simulink model "rmspec"  (Simulink 7.0)
settings: Solver=ode45  StartTime=0.0  StopTime=200  RelTol=1e-3
undefined symbols (not defined in the file): pfb_coeff_gen_calc
libraries: xbsIndex_r4 x3092, casper_library x230, xps_library x24
(part 32 of 33)

== system rmspec/pfb/fft_wideband_real1/fft_biplex_real_4x0/biplex_core/fft_stage_9/butterfly_direct/twiddle/coeff_gen ==
  rst : Inport
  Counter : xbsIndex_r4/Counter  cnt_type=Free Running  cnt_to=Inf  operation=Up  start_count=0  cnt_by_val=1  arith_type=Unsigned  n_bits=8  bin_pt=0  load_pin=off  rst=on  en=off  explicit_period=on  period=1  dbl_ovrd=off  use_behavioral_HDL=off  use_rpm=off  implementation=Fabric  block_type=counter
  ROM : xbsIndex_r4/ROM  depth=256  initVector=[1 0 0.707107543945313 -0.707107543945313 0.923881530761719 -0.382682800292969 0.382682800292969 -0.923881530761719 0.980781555175781 -0.195091247558594 0.555572509765625 -0.831466674804688 0.831466674804688 -0.555572509765625 0.195091247558594 -0.980781555175781 0.995185852050781 -0.0980148315429688 0.634391784667969 -0.77301025390625 0.881919860839844 -0.471397399902344 0.290283203125 -0.956939697265625 0.956939697265625 -0.290283203125 0.471397399902344 -0.881919860839844 0.77301025390625 -0.634391784667969 0.0980148315429688 -0.995185852050781 0.998794555664063 -0.0490646362304688 0.671562194824219 -0.740951538085938 0.90399169921875 -0.427558898925781 0.336891174316406 -0.941543579101563 0.97003173828125 -0.24298095703125 0.51409912109375 -0.85772705078125 0.803207397460938 -0.595695495605469 0.146728515625 -0.989173889160156 0.989173889160156 -0.146728515625 0.595695495605469 -0.803207397460938 0.85772705078125 -0.51409912109375 0.24298095703125 -0.97003173828125 0.941543579101563 -0.336891174316406 0.427558898925781 -0.90399169921875 0.740951538085938 -0.671562194824219 0.0490646362304688 -0.998794555664063 0.999702453613281 -0.0245437622070313 0.689537048339844 -0.724250793457031 0.914207458496094 -0.405242919921875 0.359893798828125 -0.932991027832031 0.975700378417969 -0.219100952148438 0.534996032714844 -0.844856262207031 0.817581176757813 -0.5758056640625 0.17095947265625 -0.985275268554688 0.992477416992188 -0.122413635253906 0.615234375 -0.788345336914063 0.870086669921875 -0.492897033691406 0.266716003417969 -0.963775634765625 0.949531555175781 -0.313682556152344 0.449607849121094 -0.893226623535156 0.757209777832031 -0.653175354003906 0.0735626220703125 -0.997291564941406 0.997291564941406 -0.0735626220703125 0.653175354003906 -0.757209777832031 0.893226623535156 -0.449607849121094 0.313682556152344 -0.949531555175781 0.963775634765625 -0.266716003417969 0.492897033691406 -0.870086669921875 0.788345336914063 -0.615234375 0.122413635253906 -0.992477416992188 0.985275268554688 -0.17095947265625 0.5758056640625 -0.817581176757813 0.844856262207031 -0.534996032714844 0.219100952148438 -0.975700378417969 0.932991027832031 -0.359893798828125 0.405242919921875 -0.914207458496094 0.724250793457031 -0.689537048339844 0.0245437622070313 -0.999702453613281 0.999923706054688 -0.01226806640625 0.698379516601563 -0.715728759765625 0.919113159179688 -0.393989562988281 0.371315002441406 -0.928504943847656 0.978317260742188 -0.207115173339844 0.545326232910156 -0.838226318359375 0.824592590332031 -0.56573486328125 0.183036804199219 -0.983108520507813 0.993904113769531 -0.110221862792969 0.624862670898438 -0.780738830566406 0.876068115234375 -0.482185363769531 0.278518676757813 -0.960433959960938 0.95330810546875 -0.302009582519531 0.460540771484375 -0.887641906738281 0.765167236328125 -0.643829345703125 0.0858001708984375 -0.996315002441406 0.998115539550781 -0.0613174438476563 0.66241455078125 -0.749137878417969 0.898674011230469 -0.438613891601563 0.325309753417969 -0.945610046386719 0.96697998046875 -0.254867553710938 0.5035400390625 -0.863975524902344 0.79583740234375 -0.605514526367188 0.13458251953125 -0.99090576171875 0.9873046875 -0.158859252929688 0.585800170898438 -0.810455322265625 0.851356506347656 -0.524589538574219 0.231056213378906 -0.972938537597656 0.937339782714844 -0.348419189453125 0.416427612304688 -0.909164428710938 0.732650756835938 -0.68060302734375 0.03680419921875 -0.999320983886719 0.999320983886719 -0.03680419921875 0.68060302734375 -0.732650756835938 0.909164428710938 -0.416427612304688 0.348419189453125 -0.937339782714844 0.972938537597656 -0.231056213378906 0.524589538574219 -0.851356506347656 0.810455322265625 -0.585800170898438 0.158859252929688 -0.9873046875 0.99090576171875 -0.13458251953125 0.605514526367188 -0.79583740234375 0.863975524902344 -0.5035400390625 0.254867553710938 -0.96697998046875 0.945610046386719 -0.325309753417969 0.438613891601563 -0.898674011230469 0.749137878417969 ...(+646 chars)]  distributed_mem=Block RAM  rst=off  init_reg=0  en=off  latency=2  arith_type="Signed  (2's comp)"  n_bits=18  bin_pt=17  dbl_ovrd=off  optimize=Area  use_rpm=on  block_type=sprom
      settings: block_version=10.1.3
  ROM1 : xbsIndex_r4/ROM  depth=256  initVector=[0 -1 -0.707107543945313 -0.707107543945313 -0.382682800292969 -0.923881530761719 -0.923881530761719 -0.382682800292969 -0.195091247558594 -0.980781555175781 -0.831466674804688 -0.555572509765625 -0.555572509765625 -0.831466674804688 -0.980781555175781 -0.195091247558594 -0.0980148315429688 -0.995185852050781 -0.77301025390625 -0.634391784667969 -0.471397399902344 -0.881919860839844 -0.956939697265625 -0.290283203125 -0.290283203125 -0.956939697265625 -0.881919860839844 -0.471397399902344 -0.634391784667969 -0.77301025390625 -0.995185852050781 -0.0980148315429688 -0.0490646362304688 -0.998794555664063 -0.740951538085938 -0.671562194824219 -0.427558898925781 -0.90399169921875 -0.941543579101563 -0.336891174316406 -0.24298095703125 -0.97003173828125 -0.85772705078125 -0.51409912109375 -0.595695495605469 -0.803207397460938 -0.989173889160156 -0.146728515625 -0.146728515625 -0.989173889160156 -0.803207397460938 -0.595695495605469 -0.51409912109375 -0.85772705078125 -0.97003173828125 -0.24298095703125 -0.336891174316406 -0.941543579101563 -0.90399169921875 -0.427558898925781 -0.671562194824219 -0.740951538085938 -0.998794555664063 -0.0490646362304688 -0.0245437622070313 -0.999702453613281 -0.724250793457031 -0.689537048339844 -0.405242919921875 -0.914207458496094 -0.932991027832031 -0.359893798828125 -0.219100952148438 -0.975700378417969 -0.844856262207031 -0.534996032714844 -0.5758056640625 -0.817581176757813 -0.985275268554688 -0.17095947265625 -0.122413635253906 -0.992477416992188 -0.788345336914063 -0.615234375 -0.492897033691406 -0.870086669921875 -0.963775634765625 -0.266716003417969 -0.313682556152344 -0.949531555175781 -0.893226623535156 -0.449607849121094 -0.653175354003906 -0.757209777832031 -0.997291564941406 -0.0735626220703125 -0.0735626220703125 -0.997291564941406 -0.757209777832031 -0.653175354003906 -0.449607849121094 -0.893226623535156 -0.949531555175781 -0.313682556152344 -0.266716003417969 -0.963775634765625 -0.870086669921875 -0.492897033691406 -0.615234375 -0.788345336914063 -0.992477416992188 -0.122413635253906 -0.17095947265625 -0.985275268554688 -0.817581176757813 -0.5758056640625 -0.534996032714844 -0.844856262207031 -0.975700378417969 -0.219100952148438 -0.359893798828125 -0.932991027832031 -0.914207458496094 -0.405242919921875 -0.689537048339844 -0.724250793457031 -0.999702453613281 -0.0245437622070313 -0.01226806640625 -0.999923706054688 -0.715728759765625 -0.698379516601563 -0.393989562988281 -0.919113159179688 -0.928504943847656 -0.371315002441406 -0.207115173339844 -0.978317260742188 -0.838226318359375 -0.545326232910156 -0.56573486328125 -0.824592590332031 -0.983108520507813 -0.183036804199219 -0.110221862792969 -0.993904113769531 -0.780738830566406 -0.624862670898438 -0.482185363769531 -0.876068115234375 -0.960433959960938 -0.278518676757813 -0.302009582519531 -0.95330810546875 -0.887641906738281 -0.460540771484375 -0.643829345703125 -0.765167236328125 -0.996315002441406 -0.0858001708984375 -0.0613174438476563 -0.998115539550781 -0.749137878417969 -0.66241455078125 -0.438613891601563 -0.898674011230469 -0.945610046386719 -0.325309753417969 -0.254867553710938 -0.96697998046875 -0.863975524902344 -0.5035400390625 -0.605514526367188 -0.79583740234375 -0.99090576171875 -0.13458251953125 -0.158859252929688 -0.9873046875 -0.810455322265625 -0.585800170898438 -0.524589538574219 -0.851356506347656 -0.972938537597656 -0.231056213378906 -0.348419189453125 -0.937339782714844 -0.909164428710938 -0.416427612304688 -0.68060302734375 -0.732650756835938 -0.999320983886719 -0.03680419921875 -0.03680419921875 -0.999320983886719 -0.732650756835938 -0.68060302734375 -0.416427612304688 -0.909164428710938 -0.937339782714844 -0.348419189453125 -0.231056213378906 -0.972938537597656 -0.851356506347656 -0.524589538574219 -0.585800170898438 -0.810455322265625 -0.9873046875 -0.158859252929688 -0.13458251953125 -0.99090576171875 -0.79583740234375 -0.605514526367188 -0.5035400390625 -0.863975524902344 -0.96697998046875 ...(+777 chars)]  distributed_mem=Block RAM  rst=off  init_reg=0  en=off  latency=2  arith_type="Signed  (2's comp)"  n_bits=18  bin_pt=17  dbl_ovrd=off  optimize=Area  use_rpm=on  block_type=sprom
      settings: block_version=10.1.3
  Slice : xbsIndex_r4/Slice  nbits=8  boolean_output=off  mode=Upper Bit Location + Width  bit1=0  base1=MSB of Input  bit0=0  base0=LSB of Input  dbl_ovrd=off  block_type=slice
      settings: infoedit="Extracts a given range of bits from each input sample and presents it at the output.  The output type is ordinarily unsigned with binary point at zero, but can be Boolean when the slice is one bit wide.<P><P>Hardware notes: In hardware this block costs nothing."  block_version=10.1.3
  ri_to_c : casper_library/Misc/ri_to_c  SystemSampleTime=-1
  w : Outport
  wires:
  ri_to_c/1 -> w/1
  rst/1 -> Counter/1
  Counter/1 -> Slice/1
  Slice/1 -> ROM/1, ROM1/1
  ROM/1 -> ri_to_c/1
  ROM1/1 -> ri_to_c/2

== system rmspec/pfb/fft_wideband_real1/fft_biplex_real_4x0/biplex_core/fft_stage_9/butterfly_direct/twiddle/convert_of ==
  din : Inport  OutDataType=sfix(16)  OutScaling=2^0
  convert : xbsIndex_r4/Convert  arith_type="Signed  (2's comp)"  n_bits=bit_width_o  bin_pt=binary_point_o  quantization=Truncate  overflow=Wrap  latency=latency  dbl_ovrd=off  pipeline=on  block_type=convert
      settings: block_version=10.1.1
  never : xbsIndex_r4/Constant  arith_type=Boolean  const=0  n_bits=16  bin_pt=14  explicit_period=on  period=1  equ=P=C  opselect=C  inp2=PCIN>>17  opr=+  inp1=P  carry=CIN  dbl_ovrd=off  block_type=constant
  dout : Outport
  of : Outport  Port=2
  wires:
  din/1 -> convert/1
  convert/1 -> dout/1
  never/1 -> of/1

== system rmspec/pfb/fft_wideband_real1/fft_biplex_real_4x0/biplex_core/fft_stage_9/butterfly_direct/twiddle/convert_of1 ==
  din : Inport  OutDataType=sfix(16)  OutScaling=2^0
  convert : xbsIndex_r4/Convert  arith_type="Signed  (2's comp)"  n_bits=bit_width_o  bin_pt=binary_point_o  quantization=Truncate  overflow=Wrap  latency=latency  dbl_ovrd=off  pipeline=on  block_type=convert
      settings: block_version=10.1.1
  never : xbsIndex_r4/Constant  arith_type=Boolean  const=0  n_bits=16  bin_pt=14  explicit_period=on  period=1  equ=P=C  opselect=C  inp2=PCIN>>17  opr=+  inp1=P  carry=CIN  dbl_ovrd=off  block_type=constant
  dout : Outport
  of : Outport  Port=2
  wires:
  din/1 -> convert/1
  convert/1 -> dout/1
  never/1 -> of/1

== system rmspec/w_fft/fft/fft_biplex0/biplex_core/fft_stage_10/butterfly_direct/twiddle/coeff_gen ==
  rst : Inport
  Counter : xbsIndex_r4/Counter  cnt_type=Free Running  cnt_to=Inf  operation=Up  start_count=0  cnt_by_val=1  arith_type=Unsigned  n_bits=9  bin_pt=0  load_pin=off  rst=on  en=off  explicit_period=on  period=1  dbl_ovrd=off  use_behavioral_HDL=off  use_rpm=off  implementation=Fabric  block_type=counter
  ROM : xbsIndex_r4/ROM  depth=512  initVector=[1 0 0.707107543945313 -0.707107543945313 0.923881530761719 -0.382682800292969 0.382682800292969 -0.923881530761719 0.980781555175781 -0.195091247558594 0.555572509765625 -0.831466674804688 0.831466674804688 -0.555572509765625 0.195091247558594 -0.980781555175781 0.995185852050781 -0.0980148315429688 0.634391784667969 -0.77301025390625 0.881919860839844 -0.471397399902344 0.290283203125 -0.956939697265625 0.956939697265625 -0.290283203125 0.471397399902344 -0.881919860839844 0.77301025390625 -0.634391784667969 0.0980148315429688 -0.995185852050781 0.998794555664063 -0.0490646362304688 0.671562194824219 -0.740951538085938 0.90399169921875 -0.427558898925781 0.336891174316406 -0.941543579101563 0.97003173828125 -0.24298095703125 0.51409912109375 -0.85772705078125 0.803207397460938 -0.595695495605469 0.146728515625 -0.989173889160156 0.989173889160156 -0.146728515625 0.595695495605469 -0.803207397460938 0.85772705078125 -0.51409912109375 0.24298095703125 -0.97003173828125 0.941543579101563 -0.336891174316406 0.427558898925781 -0.90399169921875 0.740951538085938 -0.671562194824219 0.0490646362304688 -0.998794555664063 0.999702453613281 -0.0245437622070313 0.689537048339844 -0.724250793457031 0.914207458496094 -0.405242919921875 0.359893798828125 -0.932991027832031 0.975700378417969 -0.219100952148438 0.534996032714844 -0.844856262207031 0.817581176757813 -0.5758056640625 0.17095947265625 -0.985275268554688 0.992477416992188 -0.122413635253906 0.615234375 -0.788345336914063 0.870086669921875 -0.492897033691406 0.266716003417969 -0.963775634765625 0.949531555175781 -0.313682556152344 0.449607849121094 -0.893226623535156 0.757209777832031 -0.653175354003906 0.0735626220703125 -0.997291564941406 0.997291564941406 -0.0735626220703125 0.653175354003906 -0.757209777832031 0.893226623535156 -0.449607849121094 0.313682556152344 -0.949531555175781 0.963775634765625 -0.266716003417969 0.492897033691406 -0.870086669921875 0.788345336914063 -0.615234375 0.122413635253906 -0.992477416992188 0.985275268554688 -0.17095947265625 0.5758056640625 -0.817581176757813 0.844856262207031 -0.534996032714844 0.219100952148438 -0.975700378417969 0.932991027832031 -0.359893798828125 0.405242919921875 -0.914207458496094 0.724250793457031 -0.689537048339844 0.0245437622070313 -0.999702453613281 0.999923706054688 -0.01226806640625 0.698379516601563 -0.715728759765625 0.919113159179688 -0.393989562988281 0.371315002441406 -0.928504943847656 0.978317260742188 -0.207115173339844 0.545326232910156 -0.838226318359375 0.824592590332031 -0.56573486328125 0.183036804199219 -0.983108520507813 0.993904113769531 -0.110221862792969 0.624862670898438 -0.780738830566406 0.876068115234375 -0.482185363769531 0.278518676757813 -0.960433959960938 0.95330810546875 -0.302009582519531 0.460540771484375 -0.887641906738281 0.765167236328125 -0.643829345703125 0.0858001708984375 -0.996315002441406 0.998115539550781 -0.0613174438476563 0.66241455078125 -0.749137878417969 0.898674011230469 -0.438613891601563 0.325309753417969 -0.945610046386719 0.96697998046875 -0.254867553710938 0.5035400390625 -0.863975524902344 0.79583740234375 -0.605514526367188 0.13458251953125 -0.99090576171875 0.9873046875 -0.158859252929688 0.585800170898438 -0.810455322265625 0.851356506347656 -0.524589538574219 0.231056213378906 -0.972938537597656 0.937339782714844 -0.348419189453125 0.416427612304688 -0.909164428710938 0.732650756835938 -0.68060302734375 0.03680419921875 -0.999320983886719 0.999320983886719 -0.03680419921875 0.68060302734375 -0.732650756835938 0.909164428710938 -0.416427612304688 0.348419189453125 -0.937339782714844 0.972938537597656 -0.231056213378906 0.524589538574219 -0.851356506347656 0.810455322265625 -0.585800170898438 0.158859252929688 -0.9873046875 0.99090576171875 -0.13458251953125 0.605514526367188 -0.79583740234375 0.863975524902344 -0.5035400390625 0.254867553710938 -0.96697998046875 0.945610046386719 -0.325309753417969 0.438613891601563 -0.898674011230469 0.749137878417969 ...(+5316 chars)]  distributed_mem=Block RAM  rst=off  init_reg=0  en=off  latency=2  arith_type="Signed  (2's comp)"  n_bits=18  bin_pt=17  dbl_ovrd=off  optimize=Area  use_rpm=on  block_type=sprom
      settings: block_version=10.1.3
  ROM1 : xbsIndex_r4/ROM  depth=512  initVector=[0 -1 -0.707107543945313 -0.707107543945313 -0.382682800292969 -0.923881530761719 -0.923881530761719 -0.382682800292969 -0.195091247558594 -0.980781555175781 -0.831466674804688 -0.555572509765625 -0.555572509765625 -0.831466674804688 -0.980781555175781 -0.195091247558594 -0.0980148315429688 -0.995185852050781 -0.77301025390625 -0.634391784667969 -0.471397399902344 -0.881919860839844 -0.956939697265625 -0.290283203125 -0.290283203125 -0.956939697265625 -0.881919860839844 -0.471397399902344 -0.634391784667969 -0.77301025390625 -0.995185852050781 -0.0980148315429688 -0.0490646362304688 -0.998794555664063 -0.740951538085938 -0.671562194824219 -0.427558898925781 -0.90399169921875 -0.941543579101563 -0.336891174316406 -0.24298095703125 -0.97003173828125 -0.85772705078125 -0.51409912109375 -0.595695495605469 -0.803207397460938 -0.989173889160156 -0.146728515625 -0.146728515625 -0.989173889160156 -0.803207397460938 -0.595695495605469 -0.51409912109375 -0.85772705078125 -0.97003173828125 -0.24298095703125 -0.336891174316406 -0.941543579101563 -0.90399169921875 -0.427558898925781 -0.671562194824219 -0.740951538085938 -0.998794555664063 -0.0490646362304688 -0.0245437622070313 -0.999702453613281 -0.724250793457031 -0.689537048339844 -0.405242919921875 -0.914207458496094 -0.932991027832031 -0.359893798828125 -0.219100952148438 -0.975700378417969 -0.844856262207031 -0.534996032714844 -0.5758056640625 -0.817581176757813 -0.985275268554688 -0.17095947265625 -0.122413635253906 -0.992477416992188 -0.788345336914063 -0.615234375 -0.492897033691406 -0.870086669921875 -0.963775634765625 -0.266716003417969 -0.313682556152344 -0.949531555175781 -0.893226623535156 -0.449607849121094 -0.653175354003906 -0.757209777832031 -0.997291564941406 -0.0735626220703125 -0.0735626220703125 -0.997291564941406 -0.757209777832031 -0.653175354003906 -0.449607849121094 -0.893226623535156 -0.949531555175781 -0.313682556152344 -0.266716003417969 -0.963775634765625 -0.870086669921875 -0.492897033691406 -0.615234375 -0.788345336914063 -0.992477416992188 -0.122413635253906 -0.17095947265625 -0.985275268554688 -0.817581176757813 -0.5758056640625 -0.534996032714844 -0.844856262207031 -0.975700378417969 -0.219100952148438 -0.359893798828125 -0.932991027832031 -0.914207458496094 -0.405242919921875 -0.689537048339844 -0.724250793457031 -0.999702453613281 -0.0245437622070313 -0.01226806640625 -0.999923706054688 -0.715728759765625 -0.698379516601563 -0.393989562988281 -0.919113159179688 -0.928504943847656 -0.371315002441406 -0.207115173339844 -0.978317260742188 -0.838226318359375 -0.545326232910156 -0.56573486328125 -0.824592590332031 -0.983108520507813 -0.183036804199219 -0.110221862792969 -0.993904113769531 -0.780738830566406 -0.624862670898438 -0.482185363769531 -0.876068115234375 -0.960433959960938 -0.278518676757813 -0.302009582519531 -0.95330810546875 -0.887641906738281 -0.460540771484375 -0.643829345703125 -0.765167236328125 -0.996315002441406 -0.0858001708984375 -0.0613174438476563 -0.998115539550781 -0.749137878417969 -0.66241455078125 -0.438613891601563 -0.898674011230469 -0.945610046386719 -0.325309753417969 -0.254867553710938 -0.96697998046875 -0.863975524902344 -0.5035400390625 -0.605514526367188 -0.79583740234375 -0.99090576171875 -0.13458251953125 -0.158859252929688 -0.9873046875 -0.810455322265625 -0.585800170898438 -0.524589538574219 -0.851356506347656 -0.972938537597656 -0.231056213378906 -0.348419189453125 -0.937339782714844 -0.909164428710938 -0.416427612304688 -0.68060302734375 -0.732650756835938 -0.999320983886719 -0.03680419921875 -0.03680419921875 -0.999320983886719 -0.732650756835938 -0.68060302734375 -0.416427612304688 -0.909164428710938 -0.937339782714844 -0.348419189453125 -0.231056213378906 -0.972938537597656 -0.851356506347656 -0.524589538574219 -0.585800170898438 -0.810455322265625 -0.9873046875 -0.158859252929688 -0.13458251953125 -0.99090576171875 -0.79583740234375 -0.605514526367188 -0.5035400390625 -0.863975524902344 -0.96697998046875 ...(+5575 chars)]  distributed_mem=Block RAM  rst=off  init_reg=0  en=off  latency=2  arith_type="Signed  (2's comp)"  n_bits=18  bin_pt=17  dbl_ovrd=off  optimize=Area  use_rpm=on  block_type=sprom
      settings: block_version=10.1.3
  Slice : xbsIndex_r4/Slice  nbits=9  boolean_output=off  mode=Upper Bit Location + Width  bit1=0  base1=MSB of Input  bit0=0  base0=LSB of Input  dbl_ovrd=off  block_type=slice
      settings: infoedit="Extracts a given range of bits from each input sample and presents it at the output.  The output type is ordinarily unsigned with binary point at zero, but can be Boolean when the slice is one bit wide.<P><P>Hardware notes: In hardware this block costs nothing."  block_version=10.1.3
  ri_to_c : casper_library/Misc/ri_to_c  SystemSampleTime=-1
  w : Outport
  wires:
  ri_to_c/1 -> w/1
  rst/1 -> Counter/1
  Counter/1 -> Slice/1
  Slice/1 -> ROM/1, ROM1/1
  ROM/1 -> ri_to_c/1
  ROM1/1 -> ri_to_c/2

== system rmspec/w_fft/fft/fft_biplex0/biplex_core/fft_stage_10/butterfly_direct/twiddle/convert_of ==
  din : Inport  OutDataType=sfix(16)  OutScaling=2^0
  convert : xbsIndex_r4/Convert  arith_type="Signed  (2's comp)"  n_bits=bit_width_o  bin_pt=binary_point_o  quantization=Truncate  overflow=Wrap  latency=latency  dbl_ovrd=off  pipeline=on  block_type=convert
      settings: block_version=10.1.1
  never : xbsIndex_r4/Constant  arith_type=Boolean  const=0  n_bits=16  bin_pt=14  explicit_period=on  period=1  equ=P=C  opselect=C  inp2=PCIN>>17  opr=+  inp1=P  carry=CIN  dbl_ovrd=off  block_type=constant
  dout : Outport
  of : Outport  Port=2
  wires:
  din/1 -> convert/1
  convert/1 -> dout/1
  never/1 -> of/1

== system rmspec/w_fft/fft/fft_biplex0/biplex_core/fft_stage_10/butterfly_direct/twiddle/convert_of1 ==
  din : Inport  OutDataType=sfix(16)  OutScaling=2^0
  convert : xbsIndex_r4/Convert  arith_type="Signed  (2's comp)"  n_bits=bit_width_o  bin_pt=binary_point_o  quantization=Truncate  overflow=Wrap  latency=latency  dbl_ovrd=off  pipeline=on  block_type=convert
      settings: block_version=10.1.1
  never : xbsIndex_r4/Constant  arith_type=Boolean  const=0  n_bits=16  bin_pt=14  explicit_period=on  period=1  equ=P=C  opselect=C  inp2=PCIN>>17  opr=+  inp1=P  carry=CIN  dbl_ovrd=off  block_type=constant
  dout : Outport
  of : Outport  Port=2
  wires:
  din/1 -> convert/1
  convert/1 -> dout/1
  never/1 -> of/1

== system rmspec/w_fft/fft/fft_biplex0/biplex_core/fft_stage_3/butterfly_direct/twiddle/coeff_gen ==
  rst : Inport
  Counter : xbsIndex_r4/Counter  cnt_type=Free Running  cnt_to=Inf  operation=Up  start_count=0  cnt_by_val=1  arith_type=Unsigned  n_bits=9  bin_pt=0  load_pin=off  rst=on  en=off  explicit_period=on  period=1  dbl_ovrd=off  use_behavioral_HDL=off  use_rpm=off  implementation=Fabric  block_type=counter
  ROM : xbsIndex_r4/ROM  depth=4  initVector=[1 0 0.707107543945313 -0.707107543945313]  distributed_mem=Distributed memory  rst=off  init_reg=0  en=off  latency=2  arith_type="Signed  (2's comp)"  n_bits=18  bin_pt=17  dbl_ovrd=off  optimize=Area  use_rpm=on  block_type=sprom
      settings: block_version=10.1.3
  ROM1 : xbsIndex_r4/ROM  depth=4  initVector=[0 -1 -0.707107543945313 -0.707107543945313]  distributed_mem=Distributed memory  rst=off  init_reg=0  en=off  latency=2  arith_type="Signed  (2's comp)"  n_bits=18  bin_pt=17  dbl_ovrd=off  optimize=Area  use_rpm=on  block_type=sprom
      settings: block_version=10.1.3
  Slice : xbsIndex_r4/Slice  nbits=2  boolean_output=off  mode=Upper Bit Location + Width  bit1=0  base1=MSB of Input  bit0=0  base0=LSB of Input  dbl_ovrd=off  block_type=slice
      settings: infoedit="Extracts a given range of bits from each input sample and presents it at the output.  The output type is ordinarily unsigned with binary point at zero, but can be Boolean when the slice is one bit wide.<P><P>Hardware notes: In hardware this block costs nothing."  block_version=10.1.3
  ri_to_c : casper_library/Misc/ri_to_c  SystemSampleTime=-1
  w : Outport
  wires:
  ri_to_c/1 -> w/1
  rst/1 -> Counter/1
  Counter/1 -> Slice/1
  Slice/1 -> ROM/1, ROM1/1
  ROM/1 -> ri_to_c/1
  ROM1/1 -> ri_to_c/2

== system rmspec/w_fft/fft/fft_biplex0/biplex_core/fft_stage_3/butterfly_direct/twiddle/convert_of ==
  din : Inport  OutDataType=sfix(16)  OutScaling=2^0
  convert : xbsIndex_r4/Convert  arith_type="Signed  (2's comp)"  n_bits=bit_width_o  bin_pt=binary_point_o  quantization=Truncate  overflow=Wrap  latency=latency  dbl_ovrd=off  pipeline=on  block_type=convert
      settings: block_version=10.1.1
  never : xbsIndex_r4/Constant  arith_type=Boolean  const=0  n_bits=16  bin_pt=14  explicit_period=on  period=1  equ=P=C  opselect=C  inp2=PCIN>>17  opr=+  inp1=P  carry=CIN  dbl_ovrd=off  block_type=constant
  dout : Outport
  of : Outport  Port=2
  wires:
  din/1 -> convert/1
  convert/1 -> dout/1
  never/1 -> of/1

== system rmspec/w_fft/fft/fft_biplex0/biplex_core/fft_stage_3/butterfly_direct/twiddle/convert_of1 ==
  din : Inport  OutDataType=sfix(16)  OutScaling=2^0
  convert : xbsIndex_r4/Convert  arith_type="Signed  (2's comp)"  n_bits=bit_width_o  bin_pt=binary_point_o  quantization=Truncate  overflow=Wrap  latency=latency  dbl_ovrd=off  pipeline=on  block_type=convert
      settings: block_version=10.1.1
  never : xbsIndex_r4/Constant  arith_type=Boolean  const=0  n_bits=16  bin_pt=14  explicit_period=on  period=1  equ=P=C  opselect=C  inp2=PCIN>>17  opr=+  inp1=P  carry=CIN  dbl_ovrd=off  block_type=constant
  dout : Outport
  of : Outport  Port=2
  wires:
  din/1 -> convert/1
  convert/1 -> dout/1
  never/1 -> of/1

== system rmspec/w_fft/fft/fft_biplex0/biplex_core/fft_stage_4/butterfly_direct/twiddle/coeff_gen ==
  rst : Inport
  Counter : xbsIndex_r4/Counter  cnt_type=Free Running  cnt_to=Inf  operation=Up  start_count=0  cnt_by_val=1  arith_type=Unsigned  n_bits=9  bin_pt=0  load_pin=off  rst=on  en=off  explicit_period=on  period=1  dbl_ovrd=off  use_behavioral_HDL=off  use_rpm=off  implementation=Fabric  block_type=counter
  ROM : xbsIndex_r4/ROM  depth=8  initVector=[1 0 0.707107543945313 -0.707107543945313 0.923881530761719 -0.382682800292969 0.382682800292969 -0.923881530761719]  distributed_mem=Distributed memory  rst=off  init_reg=0  en=off  latency=2  arith_type="Signed  (2's comp)"  n_bits=18  bin_pt=17  dbl_ovrd=off  optimize=Area  use_rpm=on  block_type=sprom
      settings: block_version=10.1.3
  ROM1 : xbsIndex_r4/ROM  depth=8  initVector=[0 -1 -0.707107543945313 -0.707107543945313 -0.382682800292969 -0.923881530761719 -0.923881530761719 -0.382682800292969]  distributed_mem=Distributed memory  rst=off  init_reg=0  en=off  latency=2  arith_type="Signed  (2's comp)"  n_bits=18  bin_pt=17  dbl_ovrd=off  optimize=Area  use_rpm=on  block_type=sprom
      settings: block_version=10.1.3
  Slice : xbsIndex_r4/Slice  nbits=3  boolean_output=off  mode=Upper Bit Location + Width  bit1=0  base1=MSB of Input  bit0=0  base0=LSB of Input  dbl_ovrd=off  block_type=slice
      settings: infoedit="Extracts a given range of bits from each input sample and presents it at the output.  The output type is ordinarily unsigned with binary point at zero, but can be Boolean when the slice is one bit wide.<P><P>Hardware notes: In hardware this block costs nothing."  block_version=10.1.3
  ri_to_c : casper_library/Misc/ri_to_c  SystemSampleTime=-1
  w : Outport
  wires:
  ri_to_c/1 -> w/1
  rst/1 -> Counter/1
  Counter/1 -> Slice/1
  Slice/1 -> ROM/1, ROM1/1
  ROM/1 -> ri_to_c/1
  ROM1/1 -> ri_to_c/2

== system rmspec/w_fft/fft/fft_biplex0/biplex_core/fft_stage_4/butterfly_direct/twiddle/convert_of ==
  din : Inport  OutDataType=sfix(16)  OutScaling=2^0
  convert : xbsIndex_r4/Convert  arith_type="Signed  (2's comp)"  n_bits=bit_width_o  bin_pt=binary_point_o  quantization=Truncate  overflow=Wrap  latency=latency  dbl_ovrd=off  pipeline=on  block_type=convert
      settings: block_version=10.1.1
  never : xbsIndex_r4/Constant  arith_type=Boolean  const=0  n_bits=16  bin_pt=14  explicit_period=on  period=1  equ=P=C  opselect=C  inp2=PCIN>>17  opr=+  inp1=P  carry=CIN  dbl_ovrd=off  block_type=constant
  dout : Outport
  of : Outport  Port=2
  wires:
  din/1 -> convert/1
  convert/1 -> dout/1
  never/1 -> of/1

== system rmspec/w_fft/fft/fft_biplex0/biplex_core/fft_stage_4/butterfly_direct/twiddle/convert_of1 ==
  din : Inport  OutDataType=sfix(16)  OutScaling=2^0
  convert : xbsIndex_r4/Convert  arith_type="Signed  (2's comp)"  n_bits=bit_width_o  bin_pt=binary_point_o  quantization=Truncate  overflow=Wrap  latency=latency  dbl_ovrd=off  pipeline=on  block_type=convert
      settings: block_version=10.1.1
  never : xbsIndex_r4/Constant  arith_type=Boolean  const=0  n_bits=16  bin_pt=14  explicit_period=on  period=1  equ=P=C  opselect=C  inp2=PCIN>>17  opr=+  inp1=P  carry=CIN  dbl_ovrd=off  block_type=constant
  dout : Outport
  of : Outport  Port=2
  wires:
  din/1 -> convert/1
  convert/1 -> dout/1
  never/1 -> of/1

== system rmspec/w_fft/fft/fft_biplex0/biplex_core/fft_stage_5/butterfly_direct/twiddle/coeff_gen ==
  rst : Inport
  Counter : xbsIndex_r4/Counter  cnt_type=Free Running  cnt_to=Inf  operation=Up  start_count=0  cnt_by_val=1  arith_type=Unsigned  n_bits=9  bin_pt=0  load_pin=off  rst=on  en=off  explicit_period=on  period=1  dbl_ovrd=off  use_behavioral_HDL=off  use_rpm=off  implementation=Fabric  block_type=counter
  ROM : xbsIndex_r4/ROM  depth=16  initVector=[1 0 0.707107543945313 -0.707107543945313 0.923881530761719 -0.382682800292969 0.382682800292969 -0.923881530761719 0.980781555175781 -0.195091247558594 0.555572509765625 -0.831466674804688 0.831466674804688 -0.555572509765625 0.195091247558594 -0.980781555175781]  distributed_mem=Block RAM  rst=off  init_reg=0  en=off  latency=2  arith_type="Signed  (2's comp)"  n_bits=18  bin_pt=17  dbl_ovrd=off  optimize=Area  use_rpm=on  block_type=sprom
      settings: block_version=10.1.3
  ROM1 : xbsIndex_r4/ROM  depth=16  initVector=[0 -1 -0.707107543945313 -0.707107543945313 -0.382682800292969 -0.923881530761719 -0.923881530761719 -0.382682800292969 -0.195091247558594 -0.980781555175781 -0.831466674804688 -0.555572509765625 -0.555572509765625 -0.831466674804688 -0.980781555175781 -0.195091247558594]  distributed_mem=Block RAM  rst=off  init_reg=0  en=off  latency=2  arith_type="Signed  (2's comp)"  n_bits=18  bin_pt=17  dbl_ovrd=off  optimize=Area  use_rpm=on  block_type=sprom
      settings: block_version=10.1.3
  Slice : xbsIndex_r4/Slice  nbits=4  boolean_output=off  mode=Upper Bit Location + Width  bit1=0  base1=MSB of Input  bit0=0  base0=LSB of Input  dbl_ovrd=off  block_type=slice
      settings: infoedit="Extracts a given range of bits from each input sample and presents it at the output.  The output type is ordinarily unsigned with binary point at zero, but can be Boolean when the slice is one bit wide.<P><P>Hardware notes: In hardware this block costs nothing."  block_version=10.1.3
  ri_to_c : casper_library/Misc/ri_to_c  SystemSampleTime=-1
  w : Outport
  wires:
  ri_to_c/1 -> w/1
  rst/1 -> Counter/1
  Counter/1 -> Slice/1
  Slice/1 -> ROM/1, ROM1/1
  ROM/1 -> ri_to_c/1
  ROM1/1 -> ri_to_c/2

== system rmspec/w_fft/fft/fft_biplex0/biplex_core/fft_stage_5/butterfly_direct/twiddle/convert_of ==
  din : Inport  OutDataType=sfix(16)  OutScaling=2^0
  convert : xbsIndex_r4/Convert  arith_type="Signed  (2's comp)"  n_bits=bit_width_o  bin_pt=binary_point_o  quantization=Truncate  overflow=Wrap  latency=latency  dbl_ovrd=off  pipeline=on  block_type=convert
      settings: block_version=10.1.1
  never : xbsIndex_r4/Constant  arith_type=Boolean  const=0  n_bits=16  bin_pt=14  explicit_period=on  period=1  equ=P=C  opselect=C  inp2=PCIN>>17  opr=+  inp1=P  carry=CIN  dbl_ovrd=off  block_type=constant
  dout : Outport
  of : Outport  Port=2
  wires:
  din/1 -> convert/1
  convert/1 -> dout/1
  never/1 -> of/1

== system rmspec/w_fft/fft/fft_biplex0/biplex_core/fft_stage_5/butterfly_direct/twiddle/convert_of1 ==
  din : Inport  OutDataType=sfix(16)  OutScaling=2^0
  convert : xbsIndex_r4/Convert  arith_type="Signed  (2's comp)"  n_bits=bit_width_o  bin_pt=binary_point_o  quantization=Truncate  overflow=Wrap  latency=latency  dbl_ovrd=off  pipeline=on  block_type=convert
      settings: block_version=10.1.1
  never : xbsIndex_r4/Constant  arith_type=Boolean  const=0  n_bits=16  bin_pt=14  explicit_period=on  period=1  equ=P=C  opselect=C  inp2=PCIN>>17  opr=+  inp1=P  carry=CIN  dbl_ovrd=off  block_type=constant
  dout : Outport
  of : Outport  Port=2
  wires:
  din/1 -> convert/1
  convert/1 -> dout/1
  never/1 -> of/1

== system rmspec/w_fft/fft/fft_biplex0/biplex_core/fft_stage_6/butterfly_direct/twiddle/coeff_gen ==
  rst : Inport
  Counter : xbsIndex_r4/Counter  cnt_type=Free Running  cnt_to=Inf  operation=Up  start_count=0  cnt_by_val=1  arith_type=Unsigned  n_bits=9  bin_pt=0  load_pin=off  rst=on  en=off  explicit_period=on  period=1  dbl_ovrd=off  use_behavioral_HDL=off  use_rpm=off  implementation=Fabric  block_type=counter
  ROM : xbsIndex_r4/ROM  depth=32  initVector=[1 0 0.707107543945313 -0.707107543945313 0.923881530761719 -0.382682800292969 0.382682800292969 -0.923881530761719 0.980781555175781 -0.195091247558594 0.555572509765625 -0.831466674804688 0.831466674804688 -0.555572509765625 0.195091247558594 -0.980781555175781 0.995185852050781 -0.0980148315429688 0.634391784667969 -0.77301025390625 0.881919860839844 -0.471397399902344 0.290283203125 -0.956939697265625 0.956939697265625 -0.290283203125 0.471397399902344 -0.881919860839844 0.77301025390625 -0.634391784667969 0.0980148315429688 -0.995185852050781]  distributed_mem=Block RAM  rst=off  init_reg=0  en=off  latency=2  arith_type="Signed  (2's comp)"  n_bits=18  bin_pt=17  dbl_ovrd=off  optimize=Area  use_rpm=on  block_type=sprom
      settings: block_version=10.1.3
  ROM1 : xbsIndex_r4/ROM  depth=32  initVector=[0 -1 -0.707107543945313 -0.707107543945313 -0.382682800292969 -0.923881530761719 -0.923881530761719 -0.382682800292969 -0.195091247558594 -0.980781555175781 -0.831466674804688 -0.555572509765625 -0.555572509765625 -0.831466674804688 -0.980781555175781 -0.195091247558594 -0.0980148315429688 -0.995185852050781 -0.77301025390625 -0.634391784667969 -0.471397399902344 -0.881919860839844 -0.956939697265625 -0.290283203125 -0.290283203125 -0.956939697265625 -0.881919860839844 -0.471397399902344 -0.634391784667969 -0.77301025390625 -0.995185852050781 -0.0980148315429688]  distributed_mem=Block RAM  rst=off  init_reg=0  en=off  latency=2  arith_type="Signed  (2's comp)"  n_bits=18  bin_pt=17  dbl_ovrd=off  optimize=Area  use_rpm=on  block_type=sprom
      settings: block_version=10.1.3
  Slice : xbsIndex_r4/Slice  nbits=5  boolean_output=off  mode=Upper Bit Location + Width  bit1=0  base1=MSB of Input  bit0=0  base0=LSB of Input  dbl_ovrd=off  block_type=slice
      settings: infoedit="Extracts a given range of bits from each input sample and presents it at the output.  The output type is ordinarily unsigned with binary point at zero, but can be Boolean when the slice is one bit wide.<P><P>Hardware notes: In hardware this block costs nothing."  block_version=10.1.3
  ri_to_c : casper_library/Misc/ri_to_c  SystemSampleTime=-1
  w : Outport
  wires:
  ri_to_c/1 -> w/1
  rst/1 -> Counter/1
  Counter/1 -> Slice/1
  Slice/1 -> ROM/1, ROM1/1
  ROM/1 -> ri_to_c/1
  ROM1/1 -> ri_to_c/2

== system rmspec/w_fft/fft/fft_biplex0/biplex_core/fft_stage_6/butterfly_direct/twiddle/convert_of ==
  din : Inport  OutDataType=sfix(16)  OutScaling=2^0
  convert : xbsIndex_r4/Convert  arith_type="Signed  (2's comp)"  n_bits=bit_width_o  bin_pt=binary_point_o  quantization=Truncate  overflow=Wrap  latency=latency  dbl_ovrd=off  pipeline=on  block_type=convert
      settings: block_version=10.1.1
  never : xbsIndex_r4/Constant  arith_type=Boolean  const=0  n_bits=16  bin_pt=14  explicit_period=on  period=1  equ=P=C  opselect=C  inp2=PCIN>>17  opr=+  inp1=P  carry=CIN  dbl_ovrd=off  block_type=constant
  dout : Outport
  of : Outport  Port=2
  wires:
  din/1 -> convert/1
  convert/1 -> dout/1
  never/1 -> of/1

== system rmspec/w_fft/fft/fft_biplex0/biplex_core/fft_stage_6/butterfly_direct/twiddle/convert_of1 ==
  din : Inport  OutDataType=sfix(16)  OutScaling=2^0
  convert : xbsIndex_r4/Convert  arith_type="Signed  (2's comp)"  n_bits=bit_width_o  bin_pt=binary_point_o  quantization=Truncate  overflow=Wrap  latency=latency  dbl_ovrd=off  pipeline=on  block_type=convert
      settings: block_version=10.1.1
  never : xbsIndex_r4/Constant  arith_type=Boolean  const=0  n_bits=16  bin_pt=14  explicit_period=on  period=1  equ=P=C  opselect=C  inp2=PCIN>>17  opr=+  inp1=P  carry=CIN  dbl_ovrd=off  block_type=constant
  dout : Outport
  of : Outport  Port=2
  wires:
  din/1 -> convert/1
  convert/1 -> dout/1
  never/1 -> of/1
